simulink model "inverter_sim_shengyu"  (R2022a)
settings: Solver=FixedStepDiscrete  StartTime=0.0  StopTime=5  FixedStep=Ts  RelTol=1e-3
PreLoadFcn:
  | sim_params;
InitFcn:
  | sim_params;
values from neighbouring files (symbols this model uses):
  DEAD_TIME_US1 = 0    [sim_params.m]
  fsw = 10000    [run_simulation.m]    (also in sim_params.m)
  Ki_vd = Ki    (= 341.85)    [sim_params.m]
  Ki_vq = Ki    (= 341.85)    [sim_params.m]
  Kp_vd = Kp    (= 3.68799083448)    [sim_params.m]
  Kp_vq = Kp    (= 3.68799083448)    [sim_params.m]
  Ls = Lls+Lm    (= 0.152752)    [load_motor_params.m]    (also in sim_params.m)
  Ts = 1e-6    (= 1e-06)    [run_simulation.m]    (also in sim_params.m)
  Vref = 380    [load_control_params.m]    (also in sim_params.m)
undefined symbols (not defined in the file or in its folder): L, R
libraries: spsDiodeLib x6, slpidlib x4, eePwmGeneratorTwoLevel x2, spsGroundLib x2, spsRMSLib x2, spsDCVoltageSourceLib x2, eeTransforms x2, artemis x1, spsAsynchronousMachineSIUnitsLib x1, spsAlphaBetaZerotodq0Lib x1, eeGeneralControl x1, simulink x1
settings Model: ARTEMISmethode_block_infos=$$__separator__$$inverter_sim_shengyu/ARTEMIS Guide$$__separator__$$  Creator=thale  LastModifiedBy=thale

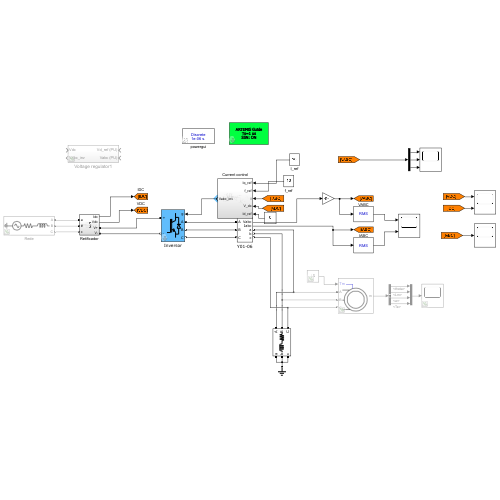
[thumbnail: Simulink's stored preview of the top-level diagram]
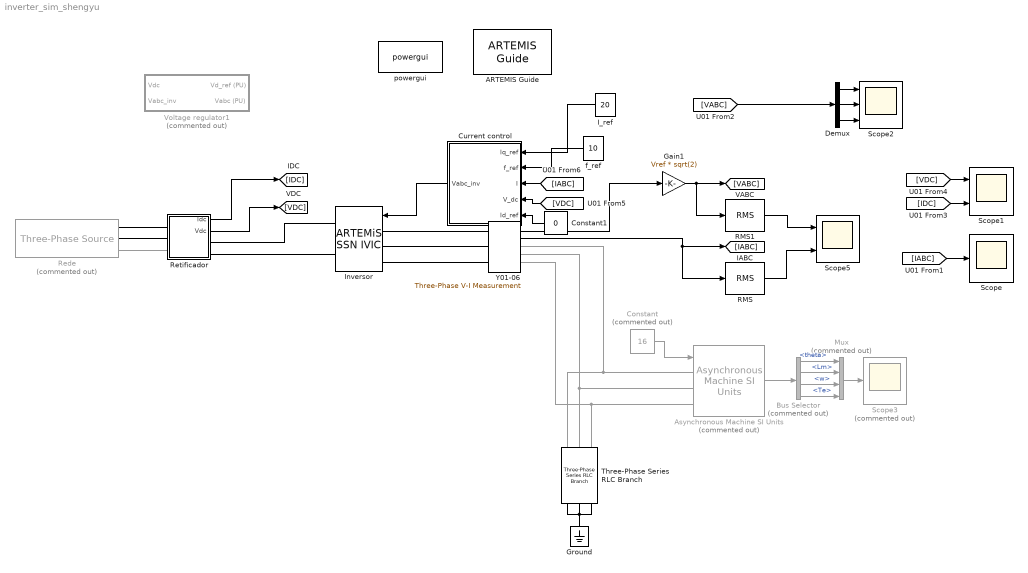
== system inverter_sim_shengyu ==
  ARTEMIS Guide : artemis/ARTEMIS/ARTEMIS Guide  Tag=art7.5  Description=New ARTEMiS block v 7.5b (R2015b+)  lock=on  Ts=Ts  ssn=on  opt=art5  dyna=off  nb_perm=4  RT_fullcomp=off  ssn_itvc=off  ssn_ivic=off  ssn_ext=off  ssn_solver=Art5  iter_type=iSWITCH and iMOV only (default)  ssn_ImpulseLoopBlockedStateUpdate=5  ssn_mov_iter_number=5  ssn_switch_iter_number=3  ssn_lu_or_ldlt=LU (more robust)  ssn_nib_type_verify=on  ssn_use_lu=on  ssn_use_ldlt=off  ssn_impulse=on  ssn_quasimpulse=off  ssn_impulse_loop=5  paraExtinctionThy=off  Thy_Impulse=on  dtc=Off  dtc_opt=normal  ao=off  simtype=off  ct_mac=off  lin_mov=off  lsp=[0.001 2]  spike_skip=Disabled  dtc_extra=1  dtc_sws=normal  dtc_pied=0.5  SPSRulesBlock=SPSRules  tre=off  ctmm=off  LF=off  dpl_type=ARTEMiS DPL  rlc_type=off  custom_type=off  para=on  ssn_full_iteration=off  ssn_init_cond=block only
  Asynchronous Machine SI Units : spsAsynchronousMachineSIUnitsLib/Asynchronous Machine SI Units  Commented=on  RotorType=Squirrel-cage  PresetModel=No  MechanicalLoad=Torque Tm  ShowDetailedParameters=on  ReferenceFrame=Rotor  Units=SI  MeasurementBus=on  NominalParameters=[3000 380 60]  VoltageRatio=1  Stator=[0.6837 0.004152]  Rotor=[0.451 0.004152]  Cage1=[0.4155 0.002066]  Cage2=[0.4168 0.0003495]  Lm=0.1486  Mechanical=[0.0120 0.008141 2]  PolePairs=2  InitialConditions=[0 0 0 0 0 0 0 0]  SimulateSaturation=off  Saturation=[14.03593122, 27.81365428, 53.79336849, 72.68890987, 97.98006896, 148.6815601, 215.7428561, 302.9841135, 428.7778367 ; 230, 322, 414, 460, 506, 552, 598, 644, 690]  LoadFlowParameters=1492000  TsPowergui=0  TsBlock=-1  IterativeModel=Trapezoidal non iterative  IterativeDiscreteModel=Trapezoidal non iterative  Pmec=1.492e+006
  Bus Selector : BusSelector  Commented=on  OutputSignals=theta,Lm,w,Te
  Constant : Constant  Commented=on  Value=16
  Constant1 : Constant  Value=0
  Current control : Subsystem
  Demux : Demux  Outputs=3
  Gain1 : Gain  Gain=Vref * sqrt(2)
  Ground : spsGroundLib/Ground  LConnTagsString=a
  I_ref : Constant  Value=20
  Inversor : ssn_inverter_model/ARTEMiS SSN IVIC  Arms=3  SnubberResistance=1e5  SnubberCapacitance=inf  Device=IGBT / Diodes  Ron=1e-3  Lon=0  ForwardVoltages=[0.8 0.8]  ForwardVoltage=0  GTOparameters=[ 10e-6 , 20e-6 ]  IGBTparameters=[ 1e-6 , 2e-6 ]*0  Measurements=None  Measurements_2=None  converterType=Rectifier
  Mux : Mux  Commented=on
  RMS : spsRMSLib/RMS  TrueRMS=off  Freq=60  RMSInit=0  Ts=Ts
  RMS1 : spsRMSLib/RMS  TrueRMS=off  Freq=60  RMSInit=0  Ts=Ts
  Rede : spsThreePhaseSourceLib/Three-Phase Source  Commented=on  InternalConnection=Yg  VoltagePhases=off  Voltage=Vref  PhaseAngle=0  Voltage_phases=[25e3 25e3 25e3]/sqrt(3)  PhaseAngles_phases=[0 -120 +120]  Frequency=60  NonIdealSource=on  SpecifyImpedance=off  Resistance=0.1  Inductance=1e-3  ShortCircuitLevel=100e6  BaseVoltage=Vref  XRratio=7  BusType=swing  Pref=10e3  Qref=0  Prefabc=[10e3, 10e3, 10e3]  Qrefabc=[0, 0, 0]  Qmin=-inf  Qmax=inf
  Retificador : Subsystem
  Scope : Scope
  Scope1 : Scope  NumInputPorts=2
  Scope2 : Scope  NumInputPorts=3
  Scope3 : Scope  Commented=on
  Scope5 : Scope  NumInputPorts=2
  Three-Phase Series RLC Branch : spsThreePhaseSeriesRLCBranchLib/Three-Phase Series RLC Branch  LConnTagsString=A|B|C  RConnTagsString=A|B|C  BranchType=RL  Resistance=R  Inductance=L  Capacitance=0  Measurements=None
  Voltage regulator1 : Subsystem  Commented=on
      settings: PortSchema="{\"entries\":[{\"content\":{\"sides\":[{\"content\":{\"connectorIds\":[\"In1\",\"In2\"]},\"type\":\"ConnectorPlacement.EquallySpacedRectSide\",\"uuid\":\"36fa6645-ebc0-40b2-a636-348de0204226\"},{\"content\":{\"connectorIds\":[\"In3\",\"Out1\"],\"side\":\"RIGHT\"},\"type\":\"ConnectorPlacement.EquallySpacedRectSide\",\"uuid\":\"6507fd83-7e4e-4d29-96e2-06567f4a5d4b\"},{\"content\":{\"connectorIds\":[],\"side\":\"TOP\"},\"type\":\"ConnectorPlacement.EquallySpacedRectSide\",\"uuid\":\"c468bd33-0f7a-476e-8b6f-3d86213f04f8\"}]},\"type\":\"ConnectorPlacement.EquallySpacedConnector\",\"uuid\":\"7f3bb63d-92f2-4b48-99c3-d8ee4ac9a4f1\"}],\"packageUris\":[\"http://schema.mathworks.com/mf0/Connector/R2020b\"],\"version\":\"1.0\"}"
  Y01-06 : spsThreePhaseVIMeasurementLib/Three-Phase V-I Measurement  VoltageMeasurement=phase-to-ground  SetLabelV=off  LabelV=Vabc  Vpu=on  VpuLL=off  CurrentMeasurement=yes  SetLabelI=off  LabelI=Iabc  Ipu=off  Pbase=100e6  Vbase=Vref  OutputType=Complex  PhasorSimulation=off  PSBequivalent=0
  f_ref : Constant  Value=10
  powergui : spspowerguiLib/powergui  Priority=1  SimulationMode=Discrete  SampleTime=Ts  frequency=60  Iterations=50  frequencyindice=0  Pbase=100e6  ErrMax=1e-4  UnitsV=kV  UnitsW=MW  buscounter=0  FunctionMessages=off  echomessages=off  EnableUseOfTLC=off  CurrentSourceSwitches=off  DisableSnubberDevices=off  DisableRonSwitches=off  DisableVfSwitches=off  DisplayEquations=off  AutomaticDiscreteSolvers=off  SolverType=Tustin/Backward Euler (TBE)  Interpol=off  ExternalGateDelay=off  methode=off  Ts=100  x0status=blocks  SPID=on  SwTol=0  HookPort=off  NonlinearTolerance=1e-4  nMaxIteration=100  ContinueOnMaxIteration=off  RestoreLinks=warning  ResistiveCurrentMeasurement=off  Frange=[0:2:500]  Ylog=off  Xlog=on  ShowGrid=off  save=off  variable=ZData  structure=0  ZoomFFT=off  StartTime=0.0  cycles=1  DisplayStyle=1  fundamental=60  FreqAxis=off  MaxFrequency=1000  frequencyindicesteady=1  RmsSteady=1  display=off
  wires:
  [IABC] -> Scope/1
  Y01-06/2 -> RMS/1, [IABC]
  [IDC] -> Scope1/2
  [VDC] -> Scope1/1
  Demux/1 -> Scope2/1
  Demux/2 -> Scope2/2
  Demux/3 -> Scope2/3
  Asynchronous Machine SI Units/1 -> Bus Selector/1
  Bus Selector/4 -> Mux/4  "<Te>"
  Bus Selector/2 -> Mux/2  "<Lm>"
  Bus Selector/3 -> Mux/3  "<w>"
  Mux/1 -> Scope3/1
  Bus Selector/1 -> Mux/1  "<theta>"
  Y01-06/1 -> Gain1/1
  RMS/1 -> Scope5/2
  Gain1/1 -> RMS1/1, [VABC]
  Current control/1(Vabc_inv) -> Inversor/1
  RMS1/1 -> Scope5/1
  [VABC] -> Demux/1
  Retificador/1(Idc) -> [IDC]
  Retificador/2(Vdc) -> [VDC]
  [VDC] -> Current control/4(V_dc)
  f_ref/1 -> Current control/2(f_ref)
  I_ref/1 -> Current control/1(Iq_ref)
  [IABC] -> Current control/3(I)
  Constant/1 -> Asynchronous Machine SI Units/1
  Constant1/1 -> Current control/5(Id_ref)
  connections:
  Inversor/LConn1 -- Y01-06/LConn1
  Inversor/LConn3 -- Y01-06/LConn3
  Inversor/LConn2 -- Y01-06/LConn2
  Asynchronous Machine SI Units/LConn3 -- Three-Phase Series RLC Branch/LConn3 -- Y01-06/RConn3
  Asynchronous Machine SI Units/LConn1 -- Three-Phase Series RLC Branch/LConn1 -- Y01-06/RConn1
  Asynchronous Machine SI Units/LConn2 -- Three-Phase Series RLC Branch/LConn2 -- Y01-06/RConn2
  Retificador/RConn1 -- Inversor/RConn1
  Retificador/LConn1 -- Rede/RConn1
  Retificador/LConn2 -- Rede/RConn2
  Rede/RConn3 -- Retificador/LConn3
  Inversor/RConn2 -- Retificador/RConn2
  Ground/LConn1 -- Three-Phase Series RLC Branch/RConn3 -- Three-Phase Series RLC Branch/RConn1 -- Three-Phase Series RLC Branch/RConn2

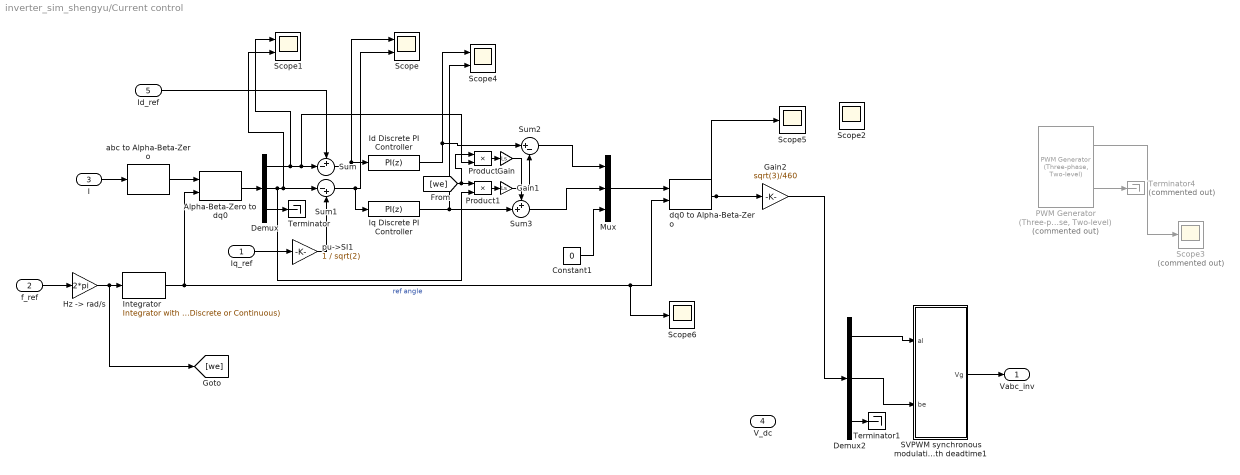
== system inverter_sim_shengyu/Current control ==
  Iq_ref : Inport
  f_ref : Inport  Port=2
  I : Inport  Port=3
  V_dc : Inport  Port=4
  Id_ref : Inport  Port=5
  Alpha-Beta-Zero to dq0 : spsAlphaBetaZerotodq0Lib/Alpha-Beta-Zero to dq0  Alignment=90 degrees behind phase A axis
      settings: SourceProductBaseCode=PS
  Constant1 : Constant  Value=0
  Demux : Demux  Outputs=3
  Demux2 : Demux  Outputs=3
  Gain : Gain  Gain=Ls
  Gain1 : Gain  Gain=Ls
  Gain2 : Gain  Gain=sqrt(3)/460
  "Hz -> rad/s" : Gain  Gain=2*pi
  Id Discrete PI Controller : slpidlib/PID Controller  Controller=PI  Form=Parallel  TimeDomain=Discrete-time  UseExternalTs=off  SampleTime=1/fsw  IntegratorMethod=Forward Euler  FilterMethod=Forward Euler  ControllerParametersSource=internal  P=Kp_vd  I=Ki_vd  UseKiTs=off  D=0  N=100  UseFilter=on  TunerSelectOption=Transfer Function Based (PID Tuner App)  InitialConditionSource=internal  InitialConditionForIntegrator=0.1  InitialConditionForFilter=0  DifferentiatorICPrevScaledInput=0  ExternalReset=none  TrackingMode=off  Kt=1  LimitOutput=off  SatLimitsSource=internal  UpperSaturationLimit=inf  LowerSaturationLimit=-1000  LinearizeAsGain=on  AntiWindupMode=none  Kb=1  POutMin=[]  POutMax=[]  IOutMin=[]  IOutMax=[]  DOutMin=[]  DOutMax=[]  NOutMin=[]  NOutMax=[]  SumOutMin=[]  SumOutMax=[]  SaturationOutMin=[]  SaturationOutMax=[]  PParamMin=[]  PParamMax=[]  IParamMin=[]  IParamMax=[]  DParamMin=[]  DParamMax=[]  NParamMin=[]  NParamMax=[]  KbParamMin=[]  KbParamMax=[]  KtParamMin=[]  KtParamMax=[]  KbOutMin=[]  KbOutMax=[]  KtOutMin=[]  KtOutMax=[]  IntegratorOutMin=[]  IntegratorOutMax=[]  FilterOutMin=[]  FilterOutMax=[]  SumI1OutMin=[]  SumI1OutMax=[]  SumI2OutMin=[]  SumI2OutMax=[]  SumI3OutMin=[]  SumI3OutMax=[]  SumI4OutMin=[]  SumI4OutMax=[]  SumDOutMin=[]  SumDOutMax=[]  DifferentiatorOutMin=[]  DifferentiatorOutMax=[]  FilterDiffOutCoefMin=[]  FilterDiffOutCoefMax=[]  ReciprocalOutMin=[]  ReciprocalOutMax=[]  SumDenOutMin=[]  SumDenOutMax=[]  SumNumOutMin=[]  SumNumOutMax=[]  DivideOutMin=[]  DivideOutMax=[]  UdiffTsProdOutMin=[]  UdiffTsProdOutMax=[]  NTsProdOutMin=[]  NTsProdOutMax=[]  UintegralTsProdOutMin=[]  UintegralTsProdOutMax=[]  UngainTsProdOutMin=[]  UngainTsProdOutMax=[]  ClampingZeroOutDataTypeStr=Inherit: Inherit via back propagation  ClampingZeroOutMin=[]  ClampingZeroOutMax=[]  FilterDenConstantOutDataTypeStr=Inherit: Inherit via back propagation  FilterDenConstantOutMin=[]  FilterDenConstantOutMax=[]  PCopyOutDataTypeStr=Inherit: Inherit via back propagation  PCopyOutMin=[]  PCopyOutMax=[]  NCopyOutDataTypeStr=Inherit: Inherit via back propagation  NCopyOutMin=[]  NCopyOutMax=[]  IntegratorContinuousStateAttributes=''  IntegratorStateMustResolveToSignalObject=off  IntegratorRTWStateStorageClass=Auto  FilterContinuousStateAttributes=''  FilterStateMustResolveToSignalObject=off  FilterRTWStateStorageClass=Auto  ParallelPVariant=InternalParameters  IdealPVariant=Disabled  IVariant=InternalParameters  DVariant=Disabled  IntegratorVariant=Discrete  SatVariant=Disabled  AWVariant=Passthrough  PCopyVariant=Disabled  TRVariant=Disabled  FdbkBlocksVariant=Forward  IdealPFdbkVariant=Disabled  SatFdbkVariant=Disabled  DerivativeFilterVariant=Disabled  NVariant=Disabled  NCopyVariant=Disabled_SignalSpec  FilterICVariant=Disabled  IntegratorICVariant=InternalICs  ExternalResetVariant=Disabled  TRSumVariant=Passthrough  SumFdbkVariant=Disabled  SumVariant=Sum_PI  TsampFilterVariant=InternalTs  TsampNgainVariant=Passthrough  TsampIntegralVariant=Passthrough  ExternalSaturationOutDataTypeStr=Inherit: Same as second input  aMode=0
  Integrator : eeGeneralControl/Integrator with Wrapped State (Discrete or Continuous)  LabelModeActiveChoice=Discrete  WrappedStateUpperValue=2*pi  WrappedStateLowerValue=0  x0=0  Ts=Ts
      settings: SourceProductBaseCode=PS
  Iq Discrete PI Controller : slpidlib/PID Controller  Controller=PI  Form=Parallel  TimeDomain=Discrete-time  UseExternalTs=off  SampleTime=1/fsw  IntegratorMethod=Forward Euler  FilterMethod=Forward Euler  ControllerParametersSource=internal  P=Kp_vq  I=Ki_vq  UseKiTs=off  D=0  N=100  UseFilter=on  TunerSelectOption=Transfer Function Based (PID Tuner App)  InitialConditionSource=internal  InitialConditionForIntegrator=1  InitialConditionForFilter=0  DifferentiatorICPrevScaledInput=0  ExternalReset=none  TrackingMode=off  Kt=1  LimitOutput=off  SatLimitsSource=internal  UpperSaturationLimit=inf  LowerSaturationLimit=-100  LinearizeAsGain=on  AntiWindupMode=none  Kb=1  POutMin=[]  POutMax=[]  IOutMin=[]  IOutMax=[]  DOutMin=[]  DOutMax=[]  NOutMin=[]  NOutMax=[]  SumOutMin=[]  SumOutMax=[]  SaturationOutMin=[]  SaturationOutMax=[]  PParamMin=[]  PParamMax=[]  IParamMin=[]  IParamMax=[]  DParamMin=[]  DParamMax=[]  NParamMin=[]  NParamMax=[]  KbParamMin=[]  KbParamMax=[]  KtParamMin=[]  KtParamMax=[]  KbOutMin=[]  KbOutMax=[]  KtOutMin=[]  KtOutMax=[]  IntegratorOutMin=[]  IntegratorOutMax=[]  FilterOutMin=[]  FilterOutMax=[]  SumI1OutMin=[]  SumI1OutMax=[]  SumI2OutMin=[]  SumI2OutMax=[]  SumI3OutMin=[]  SumI3OutMax=[]  SumI4OutMin=[]  SumI4OutMax=[]  SumDOutMin=[]  SumDOutMax=[]  DifferentiatorOutMin=[]  DifferentiatorOutMax=[]  FilterDiffOutCoefMin=[]  FilterDiffOutCoefMax=[]  ReciprocalOutMin=[]  ReciprocalOutMax=[]  SumDenOutMin=[]  SumDenOutMax=[]  SumNumOutMin=[]  SumNumOutMax=[]  DivideOutMin=[]  DivideOutMax=[]  UdiffTsProdOutMin=[]  UdiffTsProdOutMax=[]  NTsProdOutMin=[]  NTsProdOutMax=[]  UintegralTsProdOutMin=[]  UintegralTsProdOutMax=[]  UngainTsProdOutMin=[]  UngainTsProdOutMax=[]  ClampingZeroOutDataTypeStr=Inherit: Inherit via back propagation  ClampingZeroOutMin=[]  ClampingZeroOutMax=[]  FilterDenConstantOutDataTypeStr=Inherit: Inherit via back propagation  FilterDenConstantOutMin=[]  FilterDenConstantOutMax=[]  PCopyOutDataTypeStr=Inherit: Inherit via back propagation  PCopyOutMin=[]  PCopyOutMax=[]  NCopyOutDataTypeStr=Inherit: Inherit via back propagation  NCopyOutMin=[]  NCopyOutMax=[]  IntegratorContinuousStateAttributes=''  IntegratorStateMustResolveToSignalObject=off  IntegratorRTWStateStorageClass=Auto  FilterContinuousStateAttributes=''  FilterStateMustResolveToSignalObject=off  FilterRTWStateStorageClass=Auto  ParallelPVariant=InternalParameters  IdealPVariant=Disabled  IVariant=InternalParameters  DVariant=Disabled  IntegratorVariant=Discrete  SatVariant=Disabled  AWVariant=Passthrough  PCopyVariant=Disabled  TRVariant=Disabled  FdbkBlocksVariant=Forward  IdealPFdbkVariant=Disabled  SatFdbkVariant=Disabled  DerivativeFilterVariant=Disabled  NVariant=Disabled  NCopyVariant=Disabled_SignalSpec  FilterICVariant=Disabled  IntegratorICVariant=InternalICs  ExternalResetVariant=Disabled  TRSumVariant=Passthrough  SumFdbkVariant=Disabled  SumVariant=Sum_PI  TsampFilterVariant=InternalTs  TsampNgainVariant=Passthrough  TsampIntegralVariant=Passthrough  ExternalSaturationOutDataTypeStr=Inherit: Same as second input  aMode=0
  Mux : Mux  Inputs=3
  "PWM Generator (Three-phase, Two-level)" : eePwmGeneratorTwoLevel/PWM Generator (Three-phase, Two-level)  Commented=on  PWMMode=Continuous PWM (CPWM)  CPWMMode=SPWM: sinusoidal PWM  DPWMMode=60 DPWM: 60 degree discontinuous PWM  fsw=fsw  Ts=Ts
      settings: SourceProductBaseCode=PS
  Product : Product
  Product1 : Product
  SVPWM synchronous modulation with deadtime1 : Subsystem
  Scope : Scope  NumInputPorts=2
  Scope1 : Scope  NumInputPorts=2
  Scope2 : Scope
  Scope3 : Scope  Commented=on
  Scope4 : Scope  NumInputPorts=2
  Scope5 : Scope
  Scope6 : Scope
  Sum : Sum  Inputs=+-|
  Sum1 : Sum  Inputs=|-+
  Sum2 : Sum  Inputs=|+-
  Sum3 : Sum  Inputs=++|
  Terminator : Terminator
  Terminator1 : Terminator
  Terminator4 : Terminator  Commented=on
  abc to Alpha-Beta-Zero : spsabctoAlphaBetaZeroLib/abc to Alpha-Beta-Zero
      settings: SourceProductBaseCode=PS
  dq0 to Alpha-Beta-Zero : spsdq0toAlphaBetaZeroLib/dq0 to Alpha-Beta-Zero  Alignment=90 degrees behind phase A axis
      settings: SourceProductBaseCode=PS
  pu->SI1 : Gain  Gain=1 / sqrt(2)
  Vabc_inv : Outport
  wires:
  abc to Alpha-Beta-Zero/1 -> Alpha-Beta-Zero to dq0/1
  I/1 -> abc to Alpha-Beta-Zero/1
  Alpha-Beta-Zero to dq0/1 -> Demux/1
  Demux/3 -> Terminator/1
  Demux/1 -> Scope1/1, Product/2, Sum/2
  Demux/2 -> Sum1/1, Scope1/2, Product1/2
  Id_ref/1 -> Sum/1
  Sum/1 -> Scope/1, Id Discrete PI Controller/1
  Sum1/1 -> Scope/2, Iq Discrete PI Controller/1
  Constant1/1 -> Mux/3
  Mux/1 -> dq0 to Alpha-Beta-Zero/1
  f_ref/1 -> "Hz -> rad/s"/1
  "Hz -> rad/s"/1 -> [we], Integrator/1
  Integrator/1 -> Alpha-Beta-Zero to dq0/2, dq0 to Alpha-Beta-Zero/2, Scope6/1  "ref angle"
  "PWM Generator (Three-phase, Two-level)"/2 -> Terminator4/1
  "PWM Generator (Three-phase, Two-level)"/1 -> Scope3/1
  Iq_ref/1 -> pu->SI1/1
  pu->SI1/1 -> Sum1/2
  Iq Discrete PI Controller/1 -> Sum3/2, Scope4/2
  Id Discrete PI Controller/1 -> Scope4/1, Sum2/1
  Sum2/1 -> Mux/1
  Sum3/1 -> Mux/2
  [we] -> Product/1, Product1/1
  Product/1 -> Gain/1
  Gain/1 -> Sum3/1
  Product1/1 -> Gain1/1
  Gain1/1 -> Sum2/2
  SVPWM synchronous modulation with deadtime1/1(Vg) -> Vabc_inv/1
  Demux2/2 -> SVPWM synchronous modulation with deadtime1/2(be)
  Demux2/3 -> Terminator1/1
  Demux2/1 -> SVPWM synchronous modulation with deadtime1/1(al)
  dq0 to Alpha-Beta-Zero/1 -> Scope5/1, Gain2/1
  Gain2/1 -> Demux2/1

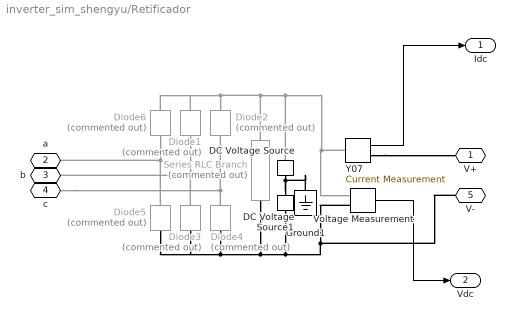
== system inverter_sim_shengyu/Retificador ==
  DC Voltage Source : spsDCVoltageSourceLib/DC Voltage Source  Amplitude=230  Measurements=None
  DC Voltage Source1 : spsDCVoltageSourceLib/DC Voltage Source  Amplitude=230  Measurements=None
  Diode{1..6} (6 alike) : spsDiodeLib/Diode  Commented=on  Ron=0.001  Lon=0  Vf=0.8  IC=0  UseSnubber=0  Rs=1e5  Cs=inf  Measurements=off
  Ground1 : spsGroundLib/Ground  LConnTagsString=a
  Series RLC Branch : spsSeriesRLCBranchLib/Series RLC Branch  Commented=on  LConnTagsString=__new0  RConnTagsString=__new0  BranchType=RC  Resistance=30e-3  Inductance=1e-3  SetiL0=off  InitialCurrent=0  Capacitance=330e-6  Setx0=off  InitialVoltage=0  Measurements=None
  Voltage Measurement : spsVoltageMeasurementLib/Voltage Measurement  PhasorSimulation=off  OutputType=Complex  PSBequivalent=0
  Y07 : spsCurrentMeasurementLib/Current Measurement  PhasorSimulation=off  OutputType=Complex  PSBequivalent=0
  V+ : PMIOPort  Side=Right
  a : PMIOPort  Port=2  Side=Left
  b : PMIOPort  Port=3  Side=Left
  c : PMIOPort  Port=4  Side=Left
  V- : PMIOPort  Port=5  Side=Right
  Idc : Outport
  Vdc : Outport  Port=2
  wires:
  Y07/1 -> Idc/1
  Voltage Measurement/1 -> Vdc/1
  connections:
  Series RLC Branch/RConn1 -- DC Voltage Source/RConn1 -- Y07/LConn1 -- Voltage Measurement/LConn1 -- Diode6/RConn1 -- Diode1/RConn1 -- Diode2/RConn1
  Diode4/RConn1 -- c/RConn1 -- Diode2/LConn1
  Diode3/RConn1 -- b/RConn1 -- Diode1/LConn1
  Series RLC Branch/LConn1 -- Diode5/LConn1 -- Diode3/LConn1 -- Diode4/LConn1 -- DC Voltage Source1/LConn1 -- V-/RConn1 -- Voltage Measurement/LConn2
  Diode5/RConn1 -- a/RConn1 -- Diode6/LConn1
  Y07/RConn1 -- V+/RConn1
  Ground1/LConn1 -- DC Voltage Source/LConn1 -- DC Voltage Source1/RConn1

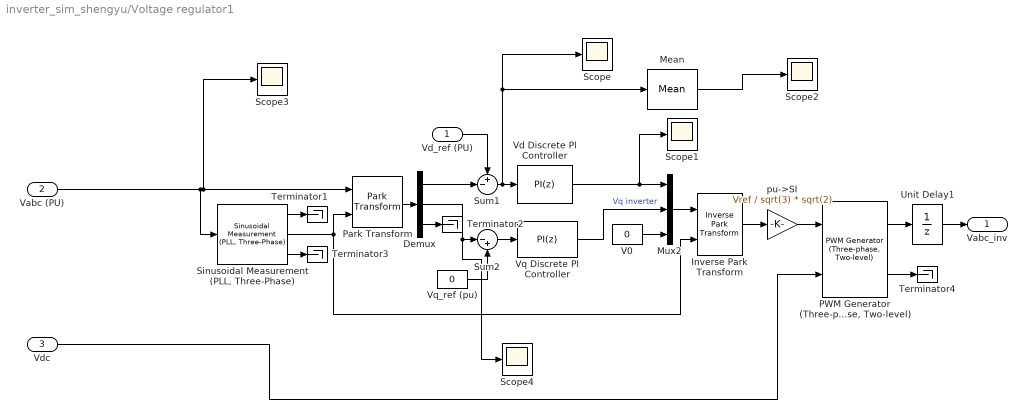
== system inverter_sim_shengyu/Voltage regulator1 ==
  Vd_ref (PU) : Inport
  Vabc (PU) : Inport  Port=2
  Vdc : Inport  Port=3
  Demux : Demux  Outputs=3
  Inverse Park Transform : eeTransforms/Inverse Park Transform  AxisAlignment=Q-axis  PowerInvariant=off
  Mean : spsMeanLib/Mean  Freq=60  Vinit=0  Ts=Ts
  Mux2 : Mux  Inputs=3
  "PWM Generator (Three-phase, Two-level)" : eePwmGeneratorTwoLevel/PWM Generator (Three-phase, Two-level)  PWMMode=Continuous PWM (CPWM)  CPWMMode=SPWM: sinusoidal PWM  DPWMMode=60 DPWM: 60 degree discontinuous PWM  fsw=fsw  Ts=Ts
      settings: SourceProductBaseCode=PS
  Park Transform : eeTransforms/Park Transform  AxisAlignment=Q-axis  PowerInvariant=off
  Scope{,1..4} (5 alike) : Scope
  "Sinusoidal Measurement (PLL, Three-Phase)" : eeSinusoidalMeasurement/Sinusoidal Measurement (PLL, Three-Phase)  Kp_LF=180  Ki_LF=3200  F0=60  Theta0=0  Ts=Ts
      settings: SourceProductBaseCode=PS
  Sum1 : Sum  Inputs=+-|  InputSameDT=on  SaturateOnIntegerOverflow=on  OutDataTypeStr=Inherit: Same as first input
  Sum2 : Sum  Inputs=|-+  InputSameDT=on  SaturateOnIntegerOverflow=on  OutDataTypeStr=Inherit: Same as first input
  Terminator{1..4} (4 alike) : Terminator
  Unit Delay1 : UnitDelay  SampleTime=Ts  HasFrameUpgradeWarning=on
  V0 : Constant  Value=0
  Vd Discrete PI Controller : slpidlib/PID Controller  Controller=PI  Form=Parallel  TimeDomain=Discrete-time  UseExternalTs=off  SampleTime=Ts  IntegratorMethod=Forward Euler  FilterMethod=Forward Euler  ControllerParametersSource=internal  P=Kp_vd  I=Ki_vd  UseKiTs=off  D=0  N=100  UseFilter=on  TunerSelectOption=Transfer Function Based (PID Tuner App)  InitialConditionSource=internal  InitialConditionForIntegrator=0.62  InitialConditionForFilter=0  DifferentiatorICPrevScaledInput=0  ExternalReset=none  TrackingMode=off  Kt=1  LimitOutput=on  SatLimitsSource=internal  UpperSaturationLimit=inf  LowerSaturationLimit=0  LinearizeAsGain=on  AntiWindupMode=none  Kb=1  POutMin=[]  POutMax=[]  IOutMin=[]  IOutMax=[]  DOutMin=[]  DOutMax=[]  NOutMin=[]  NOutMax=[]  SumOutMin=[]  SumOutMax=[]  SaturationOutMin=[]  SaturationOutMax=[]  PParamMin=[]  PParamMax=[]  IParamMin=[]  IParamMax=[]  DParamMin=[]  DParamMax=[]  NParamMin=[]  NParamMax=[]  KbParamMin=[]  KbParamMax=[]  KtParamMin=[]  KtParamMax=[]  KbOutMin=[]  KbOutMax=[]  KtOutMin=[]  KtOutMax=[]  IntegratorOutMin=[]  IntegratorOutMax=[]  FilterOutMin=[]  FilterOutMax=[]  SumI1OutMin=[]  SumI1OutMax=[]  SumI2OutMin=[]  SumI2OutMax=[]  SumI3OutMin=[]  SumI3OutMax=[]  SumI4OutMin=[]  SumI4OutMax=[]  SumDOutMin=[]  SumDOutMax=[]  DifferentiatorOutMin=[]  DifferentiatorOutMax=[]  FilterDiffOutCoefMin=[]  FilterDiffOutCoefMax=[]  ReciprocalOutMin=[]  ReciprocalOutMax=[]  SumDenOutMin=[]  SumDenOutMax=[]  SumNumOutMin=[]  SumNumOutMax=[]  DivideOutMin=[]  DivideOutMax=[]  UdiffTsProdOutMin=[]  UdiffTsProdOutMax=[]  NTsProdOutMin=[]  NTsProdOutMax=[]  UintegralTsProdOutMin=[]  UintegralTsProdOutMax=[]  UngainTsProdOutMin=[]  UngainTsProdOutMax=[]  ClampingZeroOutDataTypeStr=Inherit: Inherit via back propagation  ClampingZeroOutMin=[]  ClampingZeroOutMax=[]  FilterDenConstantOutDataTypeStr=Inherit: Inherit via back propagation  FilterDenConstantOutMin=[]  FilterDenConstantOutMax=[]  PCopyOutDataTypeStr=Inherit: Inherit via back propagation  PCopyOutMin=[]  PCopyOutMax=[]  NCopyOutDataTypeStr=Inherit: Inherit via back propagation  NCopyOutMin=[]  NCopyOutMax=[]  IntegratorContinuousStateAttributes=''  IntegratorStateMustResolveToSignalObject=off  IntegratorRTWStateStorageClass=Auto  FilterContinuousStateAttributes=''  FilterStateMustResolveToSignalObject=off  FilterRTWStateStorageClass=Auto  ParallelPVariant=InternalParameters  IdealPVariant=Disabled  IVariant=InternalParameters  DVariant=Disabled  IntegratorVariant=Discrete  SatVariant=Enabled  AWVariant=Passthrough  PCopyVariant=Disabled  TRVariant=Disabled  FdbkBlocksVariant=Forward  IdealPFdbkVariant=Disabled  SatFdbkVariant=Disabled  DerivativeFilterVariant=Disabled  NVariant=Disabled  NCopyVariant=Disabled_SignalSpec  FilterICVariant=Disabled  IntegratorICVariant=InternalICs  ExternalResetVariant=Disabled  TRSumVariant=Passthrough  SumFdbkVariant=Disabled  SumVariant=Sum_PI  TsampFilterVariant=InternalTs  TsampNgainVariant=Passthrough  TsampIntegralVariant=Passthrough  ExternalSaturationOutDataTypeStr=Inherit: Same as second input  aMode=0
  Vq Discrete PI Controller : slpidlib/PID Controller  Controller=PI  Form=Parallel  TimeDomain=Discrete-time  UseExternalTs=off  SampleTime=Ts  IntegratorMethod=Forward Euler  FilterMethod=Forward Euler  ControllerParametersSource=internal  P=Kp_vq  I=Ki_vq  UseKiTs=off  D=0  N=100  UseFilter=on  TunerSelectOption=Transfer Function Based (PID Tuner App)  InitialConditionSource=internal  InitialConditionForIntegrator=0  InitialConditionForFilter=0  DifferentiatorICPrevScaledInput=0  ExternalReset=none  TrackingMode=off  Kt=1  LimitOutput=on  SatLimitsSource=internal  UpperSaturationLimit=inf  LowerSaturationLimit=0  LinearizeAsGain=on  AntiWindupMode=none  Kb=1  POutMin=[]  POutMax=[]  IOutMin=[]  IOutMax=[]  DOutMin=[]  DOutMax=[]  NOutMin=[]  NOutMax=[]  SumOutMin=[]  SumOutMax=[]  SaturationOutMin=[]  SaturationOutMax=[]  PParamMin=[]  PParamMax=[]  IParamMin=[]  IParamMax=[]  DParamMin=[]  DParamMax=[]  NParamMin=[]  NParamMax=[]  KbParamMin=[]  KbParamMax=[]  KtParamMin=[]  KtParamMax=[]  KbOutMin=[]  KbOutMax=[]  KtOutMin=[]  KtOutMax=[]  IntegratorOutMin=[]  IntegratorOutMax=[]  FilterOutMin=[]  FilterOutMax=[]  SumI1OutMin=[]  SumI1OutMax=[]  SumI2OutMin=[]  SumI2OutMax=[]  SumI3OutMin=[]  SumI3OutMax=[]  SumI4OutMin=[]  SumI4OutMax=[]  SumDOutMin=[]  SumDOutMax=[]  DifferentiatorOutMin=[]  DifferentiatorOutMax=[]  FilterDiffOutCoefMin=[]  FilterDiffOutCoefMax=[]  ReciprocalOutMin=[]  ReciprocalOutMax=[]  SumDenOutMin=[]  SumDenOutMax=[]  SumNumOutMin=[]  SumNumOutMax=[]  DivideOutMin=[]  DivideOutMax=[]  UdiffTsProdOutMin=[]  UdiffTsProdOutMax=[]  NTsProdOutMin=[]  NTsProdOutMax=[]  UintegralTsProdOutMin=[]  UintegralTsProdOutMax=[]  UngainTsProdOutMin=[]  UngainTsProdOutMax=[]  ClampingZeroOutDataTypeStr=Inherit: Inherit via back propagation  ClampingZeroOutMin=[]  ClampingZeroOutMax=[]  FilterDenConstantOutDataTypeStr=Inherit: Inherit via back propagation  FilterDenConstantOutMin=[]  FilterDenConstantOutMax=[]  PCopyOutDataTypeStr=Inherit: Inherit via back propagation  PCopyOutMin=[]  PCopyOutMax=[]  NCopyOutDataTypeStr=Inherit: Inherit via back propagation  NCopyOutMin=[]  NCopyOutMax=[]  IntegratorContinuousStateAttributes=''  IntegratorStateMustResolveToSignalObject=off  IntegratorRTWStateStorageClass=Auto  FilterContinuousStateAttributes=''  FilterStateMustResolveToSignalObject=off  FilterRTWStateStorageClass=Auto  ParallelPVariant=InternalParameters  IdealPVariant=Disabled  IVariant=InternalParameters  DVariant=Disabled  IntegratorVariant=Discrete  SatVariant=Enabled  AWVariant=Passthrough  PCopyVariant=Disabled  TRVariant=Disabled  FdbkBlocksVariant=Forward  IdealPFdbkVariant=Disabled  SatFdbkVariant=Disabled  DerivativeFilterVariant=Disabled  NVariant=Disabled  NCopyVariant=Disabled_SignalSpec  FilterICVariant=Disabled  IntegratorICVariant=InternalICs  ExternalResetVariant=Disabled  TRSumVariant=Passthrough  SumFdbkVariant=Disabled  SumVariant=Sum_PI  TsampFilterVariant=InternalTs  TsampNgainVariant=Passthrough  TsampIntegralVariant=Passthrough  ExternalSaturationOutDataTypeStr=Inherit: Same as second input  aMode=0
  Vq_ref (pu) : Constant  Value=0
  pu->SI : Gain  Gain=Vref / sqrt(3) * sqrt(2)
  Vabc_inv : Outport
  wires:
  pu->SI/1 -> "PWM Generator (Three-phase, Two-level)"/1
  Unit Delay1/1 -> Vabc_inv/1
  "PWM Generator (Three-phase, Two-level)"/2 -> Terminator4/1
  "PWM Generator (Three-phase, Two-level)"/1 -> Unit Delay1/1
  Inverse Park Transform/1 -> pu->SI/1
  Vdc/1 -> "PWM Generator (Three-phase, Two-level)"/2
  "Sinusoidal Measurement (PLL, Three-Phase)"/1 -> Terminator1/1
  "Sinusoidal Measurement (PLL, Three-Phase)"/2 -> Inverse Park Transform/2, Park Transform/2
  "Sinusoidal Measurement (PLL, Three-Phase)"/3 -> Terminator3/1
  Demux/3 -> Terminator2/1
  Vd_ref (PU)/1 -> Sum1/1
  Demux/1 -> Sum1/2
  V0/1 -> Mux2/3
  Vq Discrete PI Controller/1 -> Mux2/2  "Vq inverter"
  Demux/2 -> Scope4/1, Sum2/1
  Vq_ref (pu)/1 -> Sum2/2
  Sum2/1 -> Vq Discrete PI Controller/1
  Park Transform/1 -> Demux/1
  Sum1/1 -> Scope/1, Mean/1, Vd Discrete PI Controller/1
  Mux2/1 -> Inverse Park Transform/1
  Vabc (PU)/1 -> "Sinusoidal Measurement (PLL, Three-Phase)"/1, Scope3/1, Park Transform/1
  Mean/1 -> Scope2/1
  Vd Discrete PI Controller/1 -> Scope1/1, Mux2/1

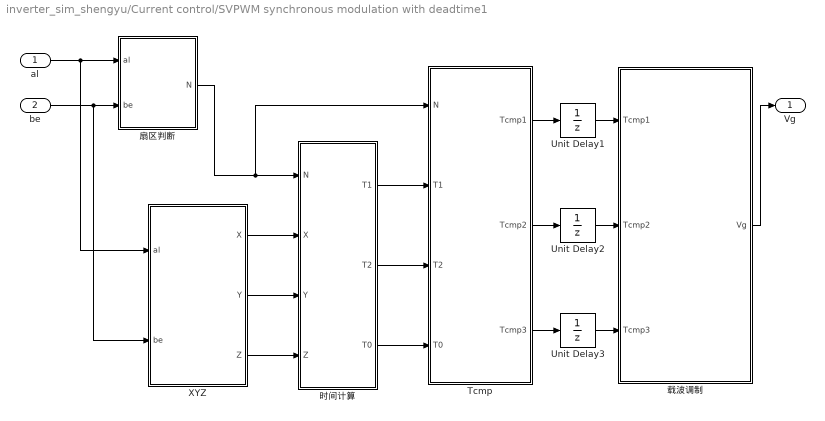
== system inverter_sim_shengyu/Current control/SVPWM synchronous modulation with deadtime1 ==
  al : Inport
  be : Inport  Port=2
  Tcmp : Subsystem
  Unit Delay1 : UnitDelay  SampleTime=Ts  HasFrameUpgradeWarning=on
  Unit Delay2 : UnitDelay  SampleTime=Ts  HasFrameUpgradeWarning=on
  Unit Delay3 : UnitDelay  SampleTime=Ts  HasFrameUpgradeWarning=on
  XYZ : Subsystem
  扇区判断 : Subsystem
  时间计算 : Subsystem
  载波调制 : Subsystem
  Vg : Outport  VectorParamsAs1DForOutWhenUnconnected=off
  wires:
  扇区判断/1(N) -> Tcmp/1(N), 时间计算/1(N)
  al/1 -> XYZ/1(al), 扇区判断/1(al)
  时间计算/2(T2) -> Tcmp/3(T2)
  XYZ/1(X) -> 时间计算/2(X)
  be/1 -> XYZ/2(be), 扇区判断/2(be)
  时间计算/1(T1) -> Tcmp/2(T1)
  XYZ/3(Z) -> 时间计算/4(Z)
  时间计算/3(T0) -> Tcmp/4(T0)
  XYZ/2(Y) -> 时间计算/3(Y)
  Tcmp/2(Tcmp2) -> Unit Delay2/1
  Tcmp/1(Tcmp1) -> Unit Delay1/1
  Tcmp/3(Tcmp3) -> Unit Delay3/1
  载波调制/1(Vg) -> Vg/1
  Unit Delay1/1 -> 载波调制/1(Tcmp1)
  Unit Delay2/1 -> 载波调制/2(Tcmp2)
  Unit Delay3/1 -> 载波调制/3(Tcmp3)

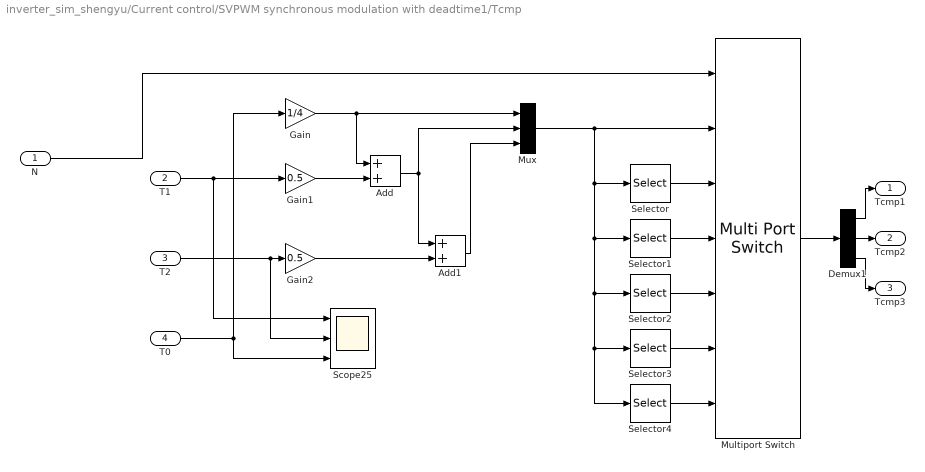
== system inverter_sim_shengyu/Current control/SVPWM synchronous modulation with deadtime1/Tcmp ==
  N : Inport
  T1 : Inport  Port=2
  T2 : Inport  Port=3
  T0 : Inport  Port=4
  Add : Sum
  Add1 : Sum
  Demux1 : Demux  Outputs=3
  Gain : Gain  Gain=1/4
  Gain1 : Gain  Gain=0.5
  Gain2 : Gain  Gain=0.5
  Multiport Switch : MultiPortSwitch  Inputs=6  DiagnosticForDefault=None  SaturateOnIntegerOverflow=off  InputSameDT=off
  Mux : Mux  Inputs=3
  Scope25 : Scope  NumInputPorts=3
  Selector : Selector  InputPortWidth=3  IndexOptions=Index vector (dialog)  Indices=[2 1 3]  OutputSizes=1
  Selector1 : Selector  InputPortWidth=3  IndexOptions=Index vector (dialog)  Indices=[3 1 2]  OutputSizes=1
  Selector2 : Selector  InputPortWidth=3  IndexOptions=Index vector (dialog)  Indices=[3 2 1]  OutputSizes=1
  Selector3 : Selector  InputPortWidth=3  IndexOptions=Index vector (dialog)  Indices=[2 3 1]  OutputSizes=1
  Selector4 : Selector  InputPortWidth=3  IndexOptions=Index vector (dialog)  Indices=[1 3 2]  OutputSizes=1
  Tcmp1 : Outport  VectorParamsAs1DForOutWhenUnconnected=off
  Tcmp2 : Outport  Port=2  VectorParamsAs1DForOutWhenUnconnected=off
  Tcmp3 : Outport  Port=3  VectorParamsAs1DForOutWhenUnconnected=off
  wires:
  Add/1 -> Add1/1, Mux/2
  Gain1/1 -> Add/2
  Gain/1 -> Mux/1, Add/1
  Multiport Switch/1 -> Demux1/1
  Gain2/1 -> Add1/2
  Mux/1 -> Selector3/1, Selector4/1, Selector2/1, Selector1/1, Selector/1, Multiport Switch/2
  T2/1 -> Scope25/2, Gain2/1
  Selector/1 -> Multiport Switch/3
  Selector4/1 -> Multiport Switch/7
  Selector3/1 -> Multiport Switch/6
  N/1 -> Multiport Switch/1
  Selector2/1 -> Multiport Switch/5
  Selector1/1 -> Multiport Switch/4
  Add1/1 -> Mux/3
  T1/1 -> Scope25/1, Gain1/1
  T0/1 -> Scope25/3, Gain/1
  Demux1/1 -> Tcmp1/1
  Demux1/2 -> Tcmp2/1
  Demux1/3 -> Tcmp3/1

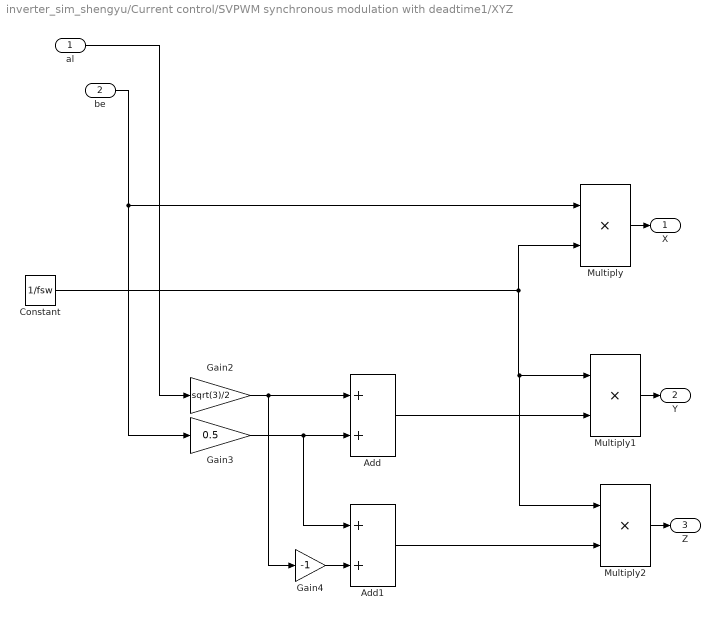
== system inverter_sim_shengyu/Current control/SVPWM synchronous modulation with deadtime1/XYZ ==
  al : Inport
  be : Inport  Port=2
  Add : Sum
  Add1 : Sum
  Constant : Constant  Value=1/fsw
  Gain2 : Gain  Gain=sqrt(3)/2
  Gain3 : Gain  Gain=0.5
  Gain4 : Gain  Gain=-1
  Multiply : Product
  Multiply1 : Product
  Multiply2 : Product
  X : Outport  VectorParamsAs1DForOutWhenUnconnected=off
  Y : Outport  Port=2  VectorParamsAs1DForOutWhenUnconnected=off
  Z : Outport  Port=3  VectorParamsAs1DForOutWhenUnconnected=off
  wires:
  Gain2/1 -> Gain4/1, Add/1
  Add/1 -> Multiply1/2
  be/1 -> Gain3/1, Multiply/1
  Gain4/1 -> Add1/2
  Multiply1/1 -> Y/1
  Constant/1 -> Multiply/2, Multiply2/1, Multiply1/1
  al/1 -> Gain2/1
  Gain3/1 -> Add1/1, Add/2
  Add1/1 -> Multiply2/2
  Multiply/1 -> X/1
  Multiply2/1 -> Z/1

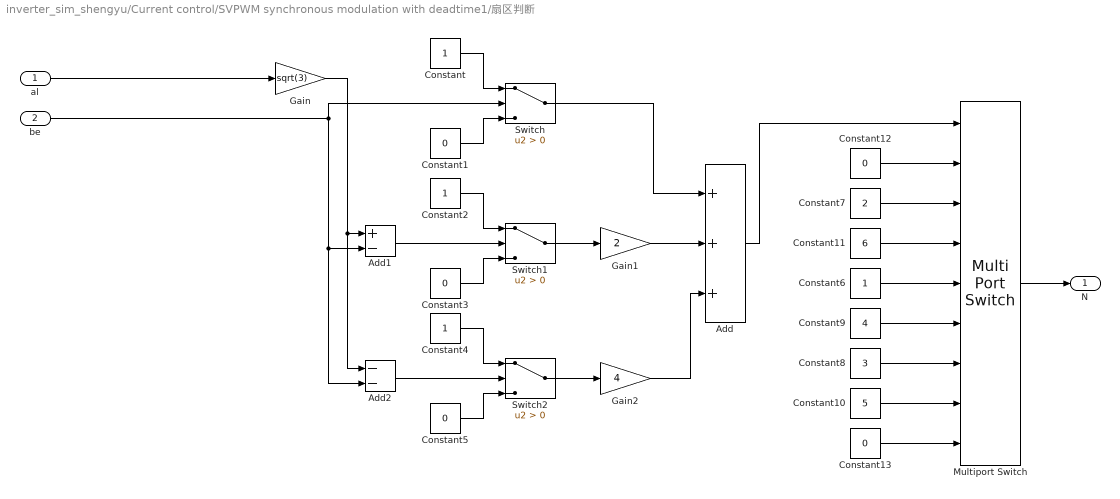
== system inverter_sim_shengyu/Current control/SVPWM synchronous modulation with deadtime1/扇区判断 ==
  al : Inport
  be : Inport  Port=2
  Add : Sum  Inputs=+++
  Add1 : Sum  Inputs=+-
  Add2 : Sum  Inputs=--
  Constant{,2,4,6} (4 alike) : Constant
  Constant{1,3,5,12..13} (5 alike) : Constant  Value=0
  Constant10 : Constant  Value=5
  Constant11 : Constant  Value=6
  Constant7 : Constant  Value=2
  Constant8 : Constant  Value=3
  Constant9 : Constant  Value=4
  Gain : Gain  Gain=sqrt(3)
  Gain1 : Gain  Gain=2
  Gain2 : Gain  Gain=4
  Multiport Switch : MultiPortSwitch  DataPortOrder=Zero-based contiguous  Inputs=8  zeroidx=on  SaturateOnIntegerOverflow=off  InputSameDT=off
  Switch : Switch  Criteria=u2 > Threshold  SaturateOnIntegerOverflow=off  InputSameDT=off
  Switch1 : Switch  Criteria=u2 > Threshold  SaturateOnIntegerOverflow=off  InputSameDT=off
  Switch2 : Switch  Criteria=u2 > Threshold  SaturateOnIntegerOverflow=off  InputSameDT=off
  N : Outport  VectorParamsAs1DForOutWhenUnconnected=off
  wires:
  Switch2/1 -> Gain2/1
  Constant1/1 -> Switch/3
  Add/1 -> Multiport Switch/1
  Constant8/1 -> Multiport Switch/7
  Constant9/1 -> Multiport Switch/6
  Gain/1 -> Add2/1, Add1/1
  Constant7/1 -> Multiport Switch/3
  Multiport Switch/1 -> N/1
  Constant10/1 -> Multiport Switch/8
  Constant3/1 -> Switch1/3
  Constant4/1 -> Switch2/1
  be/1 -> Switch/2, Add2/2, Add1/2
  Constant2/1 -> Switch1/1
  Add1/1 -> Switch1/2
  Constant11/1 -> Multiport Switch/4
  Constant5/1 -> Switch2/3
  Add2/1 -> Switch2/2
  Constant12/1 -> Multiport Switch/2
  Constant/1 -> Switch/1
  Constant13/1 -> Multiport Switch/9
  Constant6/1 -> Multiport Switch/5
  al/1 -> Gain/1
  Gain2/1 -> Add/3
  Gain1/1 -> Add/2
  Switch1/1 -> Gain1/1
  Switch/1 -> Add/1

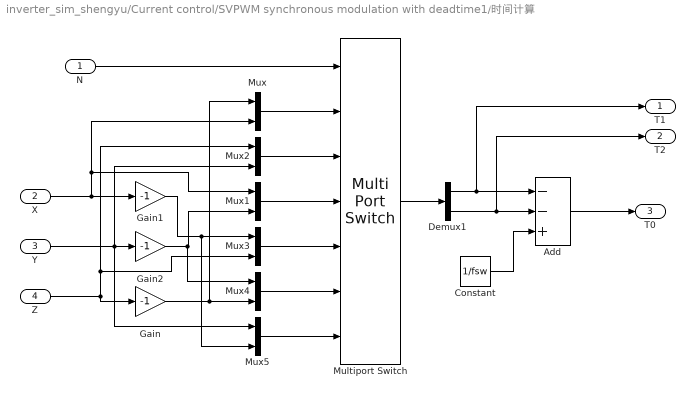
== system inverter_sim_shengyu/Current control/SVPWM synchronous modulation with deadtime1/时间计算 ==
  N : Inport
  X : Inport  Port=2
  Y : Inport  Port=3
  Z : Inport  Port=4
  Add : Sum  Inputs=--+
  Constant : Constant  Value=1/fsw
  Demux1 : Demux  Outputs=2
  Gain : Gain  Gain=-1
  Gain1 : Gain  Gain=-1
  Gain2 : Gain  Gain=-1
  Multiport Switch : MultiPortSwitch  Inputs=6  DiagnosticForDefault=None  SaturateOnIntegerOverflow=off  InputSameDT=off
  Mux{,1..5} (6 alike) : Mux  Inputs=2
  T1 : Outport  VectorParamsAs1DForOutWhenUnconnected=off
  T2 : Outport  Port=2  VectorParamsAs1DForOutWhenUnconnected=off
  T0 : Outport  Port=3  VectorParamsAs1DForOutWhenUnconnected=off
  wires:
  X/1 -> Mux1/1, Mux/2, Gain1/1
  Mux1/1 -> Multiport Switch/4
  Z/1 -> Mux3/2, Mux2/1, Gain/1
  Demux1/2 -> T2/1, Add/2
  Gain1/1 -> Mux5/2, Mux3/1
  Gain/1 -> Mux/1, Mux4/2
  Demux1/1 -> T1/1, Add/1
  Gain2/1 -> Mux4/1, Mux1/2
  Y/1 -> Mux5/1, Mux2/2, Gain2/1
  Mux/1 -> Multiport Switch/2
  Mux5/1 -> Multiport Switch/7
  Multiport Switch/1 -> Demux1/1
  Mux3/1 -> Multiport Switch/5
  Mux2/1 -> Multiport Switch/3
  Mux4/1 -> Multiport Switch/6
  N/1 -> Multiport Switch/1
  Add/1 -> T0/1
  Constant/1 -> Add/3

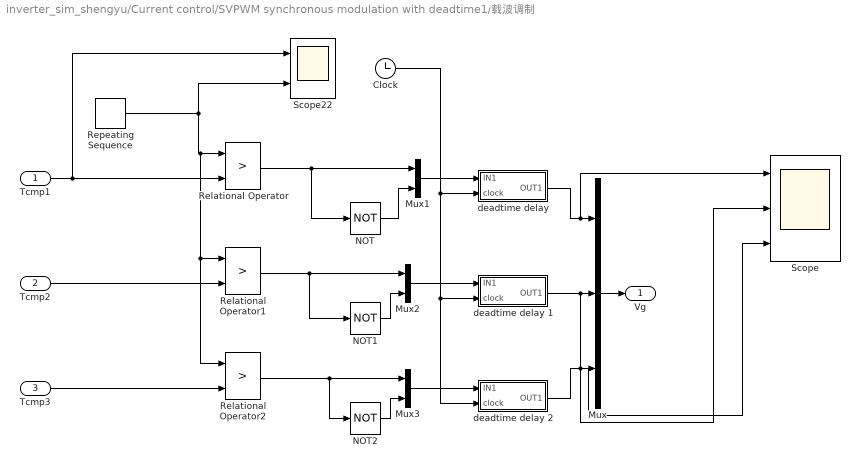
== system inverter_sim_shengyu/Current control/SVPWM synchronous modulation with deadtime1/载波调制 ==
  Tcmp1 : Inport
  Tcmp2 : Inport  Port=2
  Tcmp3 : Inport  Port=3
  Clock : Clock
  Mux : Mux  Inputs=3
  Mux1 : Mux  Inputs=2
  Mux2 : Mux  Inputs=2
  Mux3 : Mux  Inputs=2
  NOT : Logic  Operator=NOT  IconShape=distinctive  AllPortsSameDT=off  OutDataTypeStr=boolean
  NOT1 : Logic  Operator=NOT  IconShape=distinctive  AllPortsSameDT=off  OutDataTypeStr=boolean
  NOT2 : Logic  Operator=NOT  IconShape=distinctive  AllPortsSameDT=off  OutDataTypeStr=boolean
  Relational Operator : RelationalOperator  Operator=>  OutDataTypeStr=boolean  RndMeth=Simplest  InputSameDT=off
  Relational Operator1 : RelationalOperator  Operator=>  OutDataTypeStr=boolean  RndMeth=Simplest  InputSameDT=off
  Relational Operator2 : RelationalOperator  Operator=>  OutDataTypeStr=boolean  RndMeth=Simplest  InputSameDT=off
  Repeating Sequence : simulink/Sources/Repeating Sequence  rep_seq_t=[0 1/(fsw*2) 1/fsw]  rep_seq_y=[0 1/(fsw*2) 0]
  Scope : Scope  NumInputPorts=3
  Scope22 : Scope  NumInputPorts=2
  "deadtime delay " : Subsystem
  deadtime delay 1 : Subsystem
  deadtime delay 2 : Subsystem
  Vg : Outport  VectorParamsAs1DForOutWhenUnconnected=off
  wires:
  Relational Operator2/1 -> Mux3/1, NOT2/1
  Relational Operator/1 -> NOT/1, Mux1/1
  Relational Operator1/1 -> NOT1/1, Mux2/1
  Tcmp3/1 -> Relational Operator2/2
  Tcmp2/1 -> Relational Operator1/2
  Tcmp1/1 -> Relational Operator/2, Scope22/1
  Repeating Sequence/1 -> Scope22/2, Relational Operator2/1, Relational Operator1/1, Relational Operator/1
  Mux/1 -> Vg/1
  Clock/1 -> deadtime delay 2/2(clock), deadtime delay 1/2(clock), "deadtime delay "/2(clock)
  Mux1/1 -> "deadtime delay "/1(IN1)
  NOT/1 -> Mux1/2
  NOT1/1 -> Mux2/2
  Mux2/1 -> deadtime delay 1/1(IN1)
  NOT2/1 -> Mux3/2
  Mux3/1 -> deadtime delay 2/1(IN1)
  "deadtime delay "/1(OUT1) -> Scope/1, Mux/1
  deadtime delay 1/1(OUT1) -> Scope/2, Mux/2
  deadtime delay 2/1(OUT1) -> Scope/3, Mux/3

== system inverter_sim_shengyu/Current control/SVPWM synchronous modulation with deadtime1/载波调制/deadtime delay  ==
  IN1 : Inport
  clock : Inport  Port=2
  Constant : Constant
  Constant1 : Constant  Value=DEAD_TIME_US1
  Data Type Conversion1 : DataTypeConversion  OutDataTypeStr=boolean
  ON Delay : Subsystem  TreatAsAtomicUnit=on
  OUT1 : Outport
  wires:
  Data Type Conversion1/1 -> ON Delay/1(IN)
  ON Delay/1(OUT) -> OUT1/1
  Constant1/1 -> ON Delay/3(DELAY)
  clock/1 -> ON Delay/2(clock)
  IN1/1 -> Data Type Conversion1/1
  Constant/1 -> ON Delay/Enable

== system inverter_sim_shengyu/Current control/SVPWM synchronous modulation with deadtime1/载波调制/deadtime delay 1 ==
  IN1 : Inport
  clock : Inport  Port=2
  Constant : Constant
  Constant1 : Constant  Value=DEAD_TIME_US1
  Data Type Conversion1 : DataTypeConversion  OutDataTypeStr=boolean
  ON Delay : Subsystem  TreatAsAtomicUnit=on
  OUT1 : Outport
  wires:
  Data Type Conversion1/1 -> ON Delay/1(IN)
  ON Delay/1(OUT) -> OUT1/1
  Constant1/1 -> ON Delay/3(DELAY)
  clock/1 -> ON Delay/2(clock)
  IN1/1 -> Data Type Conversion1/1
  Constant/1 -> ON Delay/Enable

== system inverter_sim_shengyu/Current control/SVPWM synchronous modulation with deadtime1/载波调制/deadtime delay 2 ==
  IN1 : Inport
  clock : Inport  Port=2
  Constant : Constant
  Constant1 : Constant  Value=DEAD_TIME_US1
  Data Type Conversion1 : DataTypeConversion  OutDataTypeStr=boolean
  ON Delay : Subsystem  TreatAsAtomicUnit=on
  OUT1 : Outport
  wires:
  Data Type Conversion1/1 -> ON Delay/1(IN)
  ON Delay/1(OUT) -> OUT1/1
  Constant1/1 -> ON Delay/3(DELAY)
  clock/1 -> ON Delay/2(clock)
  IN1/1 -> Data Type Conversion1/1
  Constant/1 -> ON Delay/Enable

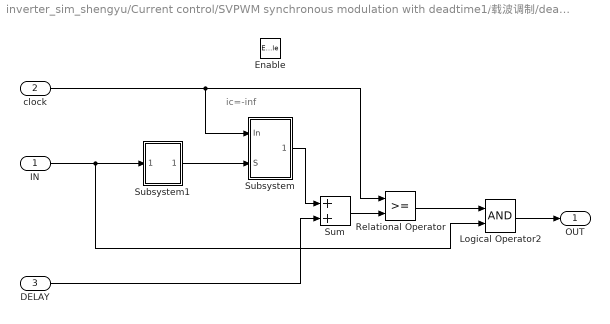
== system inverter_sim_shengyu/Current control/SVPWM synchronous modulation with deadtime1/载波调制/deadtime delay /ON Delay ==
  note: ic=-inf
  IN : Inport
  clock : Inport  Port=2
  DELAY : Inport  Port=3
  Enable : EnablePort  PropagateVarSize=During execution
  Logical Operator2 : Logic
  Relational Operator : RelationalOperator  OutDataTypeStr=boolean
  Subsystem : Subsystem
  Subsystem1 : Subsystem
  Sum : Sum  InputSameDT=on  SaturateOnIntegerOverflow=on  OutDataTypeStr=Inherit: Same as first input
  OUT : Outport
  wires:
  Subsystem/1("   ") -> Sum/1
  DELAY/1 -> Sum/2
  Sum/1 -> Relational Operator/2
  clock/1 -> Subsystem/1(In), Relational Operator/1
  Logical Operator2/1 -> OUT/1
  IN/1 -> Subsystem1/1(In1), Logical Operator2/2
  Subsystem1/1(Out) -> Subsystem/2(S)
  Relational Operator/1 -> Logical Operator2/1

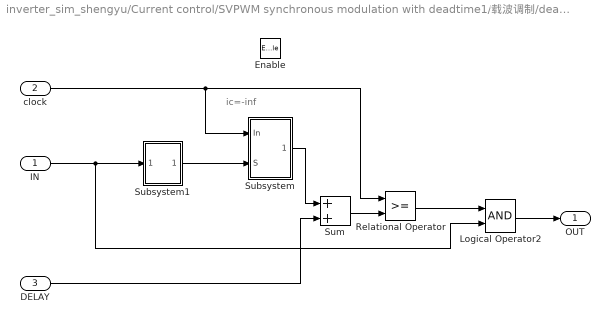
== system inverter_sim_shengyu/Current control/SVPWM synchronous modulation with deadtime1/载波调制/deadtime delay 1/ON Delay ==
  note: ic=-inf
  IN : Inport
  clock : Inport  Port=2
  DELAY : Inport  Port=3
  Enable : EnablePort  PropagateVarSize=During execution
  Logical Operator2 : Logic
  Relational Operator : RelationalOperator  OutDataTypeStr=boolean
  Subsystem : Subsystem
  Subsystem1 : Subsystem
  Sum : Sum  InputSameDT=on  SaturateOnIntegerOverflow=on  OutDataTypeStr=Inherit: Same as first input
  OUT : Outport
  wires:
  Subsystem/1("   ") -> Sum/1
  DELAY/1 -> Sum/2
  Sum/1 -> Relational Operator/2
  clock/1 -> Subsystem/1(In), Relational Operator/1
  Logical Operator2/1 -> OUT/1
  IN/1 -> Subsystem1/1(In1), Logical Operator2/2
  Subsystem1/1(Out) -> Subsystem/2(S)
  Relational Operator/1 -> Logical Operator2/1

== system inverter_sim_shengyu/Current control/SVPWM synchronous modulation with deadtime1/载波调制/deadtime delay 2/ON Delay ==
  note: ic=-inf
  IN : Inport
  clock : Inport  Port=2
  DELAY : Inport  Port=3
  Enable : EnablePort  PropagateVarSize=During execution
  Logical Operator2 : Logic
  Relational Operator : RelationalOperator  OutDataTypeStr=boolean
  Subsystem : Subsystem
  Subsystem1 : Subsystem
  Sum : Sum  InputSameDT=on  SaturateOnIntegerOverflow=on  OutDataTypeStr=Inherit: Same as first input
  OUT : Outport
  wires:
  Subsystem/1("   ") -> Sum/1
  DELAY/1 -> Sum/2
  Sum/1 -> Relational Operator/2
  clock/1 -> Subsystem/1(In), Relational Operator/1
  Logical Operator2/1 -> OUT/1
  IN/1 -> Subsystem1/1(In1), Logical Operator2/2
  Subsystem1/1(Out) -> Subsystem/2(S)
  Relational Operator/1 -> Logical Operator2/1

== system inverter_sim_shengyu/Current control/SVPWM synchronous modulation with deadtime1/载波调制/deadtime delay /ON Delay/Subsystem ==
  In : Inport
  S : Inport  Port=2
  IC=ic : Memory  InitialCondition=-1e99  InheritSampleTime=on
  Switch : Switch  Threshold=0.5
  "   " : Outport  InitialOutput=0
  wires:
  Switch/1 -> "   "/1, IC=ic/1
  S/1 -> Switch/2
  In/1 -> Switch/1
  IC=ic/1 -> Switch/3

== system inverter_sim_shengyu/Current control/SVPWM synchronous modulation with deadtime1/载波调制/deadtime delay /ON Delay/Subsystem1 ==
  In1 : Inport
  Demux : Demux  Outputs=2
      settings: DisplayOption=none
  Logical Operator1 : Logic  Operator=OR
  Memory : Memory  InheritSampleTime=on  LinearizeAsDelay=on
  NEGATIVE Edge : Subsystem  TreatAsAtomicUnit=on
  POSITIVE Edge : Subsystem  TreatAsAtomicUnit=on
  pos. edge : Constant  Value=[1 0]
  Out : Outport
  wires:
  Demux/2 -> NEGATIVE Edge/Enable
  Logical Operator1/1 -> Out/1
  Demux/1 -> POSITIVE Edge/Enable
  In1/1 -> POSITIVE Edge/1(IN), NEGATIVE Edge/1(IN), Memory/1
  pos. edge/1 -> Demux/1
  Memory/1 -> POSITIVE Edge/2(IN previous), NEGATIVE Edge/2(IN previous)
  POSITIVE Edge/1(OUT) -> Logical Operator1/1
  NEGATIVE Edge/1(OUT) -> Logical Operator1/2

== system inverter_sim_shengyu/Current control/SVPWM synchronous modulation with deadtime1/载波调制/deadtime delay 1/ON Delay/Subsystem ==
  In : Inport
  S : Inport  Port=2
  IC=ic : Memory  InitialCondition=-1e99  InheritSampleTime=on
  Switch : Switch  Threshold=0.5
  "   " : Outport  InitialOutput=0
  wires:
  Switch/1 -> "   "/1, IC=ic/1
  S/1 -> Switch/2
  In/1 -> Switch/1
  IC=ic/1 -> Switch/3

== system inverter_sim_shengyu/Current control/SVPWM synchronous modulation with deadtime1/载波调制/deadtime delay 1/ON Delay/Subsystem1 ==
  In1 : Inport
  Demux : Demux  Outputs=2
      settings: DisplayOption=none
  Logical Operator1 : Logic  Operator=OR
  Memory : Memory  InheritSampleTime=on  LinearizeAsDelay=on
  NEGATIVE Edge : Subsystem  TreatAsAtomicUnit=on
  POSITIVE Edge : Subsystem  TreatAsAtomicUnit=on
  pos. edge : Constant  Value=[1 0]
  Out : Outport
  wires:
  Demux/2 -> NEGATIVE Edge/Enable
  Logical Operator1/1 -> Out/1
  Demux/1 -> POSITIVE Edge/Enable
  In1/1 -> POSITIVE Edge/1(IN), NEGATIVE Edge/1(IN), Memory/1
  pos. edge/1 -> Demux/1
  Memory/1 -> POSITIVE Edge/2(IN previous), NEGATIVE Edge/2(IN previous)
  POSITIVE Edge/1(OUT) -> Logical Operator1/1
  NEGATIVE Edge/1(OUT) -> Logical Operator1/2

== system inverter_sim_shengyu/Current control/SVPWM synchronous modulation with deadtime1/载波调制/deadtime delay 2/ON Delay/Subsystem ==
  In : Inport
  S : Inport  Port=2
  IC=ic : Memory  InitialCondition=-1e99  InheritSampleTime=on
  Switch : Switch  Threshold=0.5
  "   " : Outport  InitialOutput=0
  wires:
  Switch/1 -> "   "/1, IC=ic/1
  S/1 -> Switch/2
  In/1 -> Switch/1
  IC=ic/1 -> Switch/3

== system inverter_sim_shengyu/Current control/SVPWM synchronous modulation with deadtime1/载波调制/deadtime delay 2/ON Delay/Subsystem1 ==
  In1 : Inport
  Demux : Demux  Outputs=2
      settings: DisplayOption=none
  Logical Operator1 : Logic  Operator=OR
  Memory : Memory  InheritSampleTime=on  LinearizeAsDelay=on
  NEGATIVE Edge : Subsystem  TreatAsAtomicUnit=on
  POSITIVE Edge : Subsystem  TreatAsAtomicUnit=on
  pos. edge : Constant  Value=[1 0]
  Out : Outport
  wires:
  Demux/2 -> NEGATIVE Edge/Enable
  Logical Operator1/1 -> Out/1
  Demux/1 -> POSITIVE Edge/Enable
  In1/1 -> POSITIVE Edge/1(IN), NEGATIVE Edge/1(IN), Memory/1
  pos. edge/1 -> Demux/1
  Memory/1 -> POSITIVE Edge/2(IN previous), NEGATIVE Edge/2(IN previous)
  POSITIVE Edge/1(OUT) -> Logical Operator1/1
  NEGATIVE Edge/1(OUT) -> Logical Operator1/2

== system inverter_sim_shengyu/Current control/SVPWM synchronous modulation with deadtime1/载波调制/deadtime delay /ON Delay/Subsystem1/NEGATIVE Edge ==
  IN : Inport
  IN previous : Inport  Port=2
  Enable : EnablePort  PropagateVarSize=During execution
  Relational Operator1 : RelationalOperator  Operator=>
  OUT : Outport
  wires:
  Relational Operator1/1 -> OUT/1
  IN previous/1 -> Relational Operator1/1
  IN/1 -> Relational Operator1/2

== system inverter_sim_shengyu/Current control/SVPWM synchronous modulation with deadtime1/载波调制/deadtime delay /ON Delay/Subsystem1/POSITIVE Edge ==
  IN : Inport
  IN previous : Inport  Port=2
  Enable : EnablePort  PropagateVarSize=During execution
  Relational Operator1 : RelationalOperator  Operator=>
  OUT : Outport
  wires:
  Relational Operator1/1 -> OUT/1
  IN previous/1 -> Relational Operator1/2
  IN/1 -> Relational Operator1/1

== system inverter_sim_shengyu/Current control/SVPWM synchronous modulation with deadtime1/载波调制/deadtime delay 1/ON Delay/Subsystem1/NEGATIVE Edge ==
  IN : Inport
  IN previous : Inport  Port=2
  Enable : EnablePort  PropagateVarSize=During execution
  Relational Operator1 : RelationalOperator  Operator=>
  OUT : Outport
  wires:
  Relational Operator1/1 -> OUT/1
  IN previous/1 -> Relational Operator1/1
  IN/1 -> Relational Operator1/2

== system inverter_sim_shengyu/Current control/SVPWM synchronous modulation with deadtime1/载波调制/deadtime delay 1/ON Delay/Subsystem1/POSITIVE Edge ==
  IN : Inport
  IN previous : Inport  Port=2
  Enable : EnablePort  PropagateVarSize=During execution
  Relational Operator1 : RelationalOperator  Operator=>
  OUT : Outport
  wires:
  Relational Operator1/1 -> OUT/1
  IN previous/1 -> Relational Operator1/2
  IN/1 -> Relational Operator1/1

== system inverter_sim_shengyu/Current control/SVPWM synchronous modulation with deadtime1/载波调制/deadtime delay 2/ON Delay/Subsystem1/NEGATIVE Edge ==
  IN : Inport
  IN previous : Inport  Port=2
  Enable : EnablePort  PropagateVarSize=During execution
  Relational Operator1 : RelationalOperator  Operator=>
  OUT : Outport
  wires:
  Relational Operator1/1 -> OUT/1
  IN previous/1 -> Relational Operator1/1
  IN/1 -> Relational Operator1/2

== system inverter_sim_shengyu/Current control/SVPWM synchronous modulation with deadtime1/载波调制/deadtime delay 2/ON Delay/Subsystem1/POSITIVE Edge ==
  IN : Inport
  IN previous : Inport  Port=2
  Enable : EnablePort  PropagateVarSize=During execution
  Relational Operator1 : RelationalOperator  Operator=>
  OUT : Outport
  wires:
  Relational Operator1/1 -> OUT/1
  IN previous/1 -> Relational Operator1/2
  IN/1 -> Relational Operator1/1
